simulink model "s2dot2_47_zidongfuweijishuqi"  (R2023b)
settings: Solver=VariableStepAuto  StartTime=0.0  StopTime=10.0  RelTol=1e-3
settings Model: Creator=lxj  LastModifiedBy=lxj

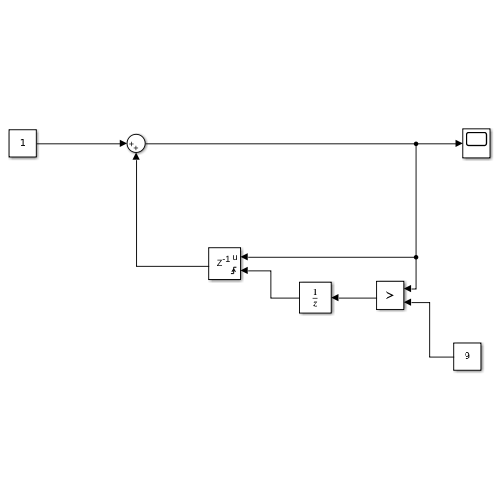
[thumbnail: Simulink's stored preview of the top-level diagram]
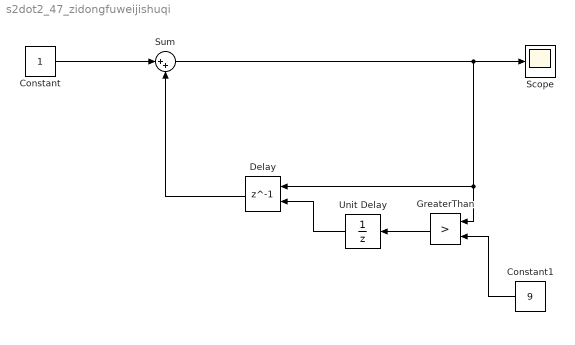
== system s2dot2_47_zidongfuweijishuqi ==
  Constant : Constant
  Constant1 : Constant  Value=9
  Delay : Delay  DelayLength=1  InitialCondition=0  ExternalReset=Rising
      settings: InputPortMap=u0,r5
  GreaterThan : RelationalOperator  Operator=>  OutDataTypeStr=boolean  RndMeth=Simplest  InputSameDT=off
  Scope : Scope
  Sum : Sum  Inputs=|++
  Unit Delay : UnitDelay  SampleTime=-1  HasFrameUpgradeWarning=on
  wires:
  Constant/1 -> Sum/1
  Sum/1 -> Delay/1, GreaterThan/1, Scope/1
  Delay/1 -> Sum/2
  Constant1/1 -> GreaterThan/2
  GreaterThan/1 -> Unit Delay/1
  Unit Delay/1 -> Delay/2
